simulink model "new_photovoltaic_battery_commonload"  (R2022b)
settings: Solver=FixedStepAuto  StartTime=0  StopTime=2.4  FixedStep=2e-5  RelTol=1e-3
undefined symbols (not defined in the file): Acid, Lead, sigbuilder_block
libraries: spsMeanLib x22, spsVoltageMeasurementLib x19, spsCurrentMeasurementLib x16, spsGroundLib x15, spsIdealSwitchLib x12, spsSeriesRLCLoadLib x12, spsSeriesRLCBranchLib x5, simulink x4, spsThreePhaseVIMeasurementLib x4, spsThreePhaseSeriesRLCBranchLib x2, spsThreePhaseBreakerLib x2, slpidlib x2
(part 2 of 2)

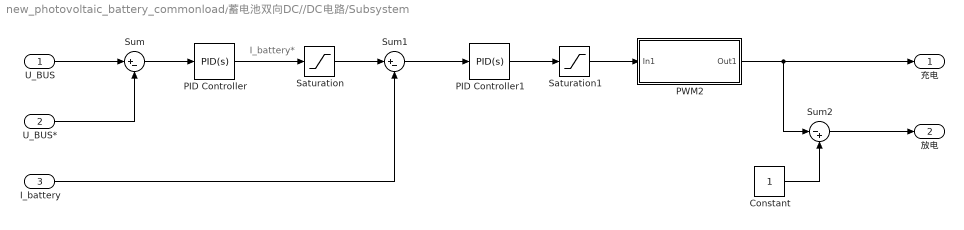
== system new_photovoltaic_battery_commonload/蓄电池双向DC//DC电路/Subsystem ==
  note: I_battery*
  U_BUS : Inport
  U_BUS* : Inport  Port=2
  I_battery : Inport  Port=3
  Constant : Constant
  PID Controller : slpidlib/PID Controller  Controller=PID  Form=Parallel  TimeDomain=Continuous-time  UseExternalTs=off  SampleTime=-1  IntegratorMethod=Forward Euler  FilterMethod=Forward Euler  ControllerParametersSource=internal  P=0.1  I=1  UseKiTs=off  D=0  N=100  UseFilter=on  TunerSelectOption=Transfer Function Based (PID Tuner App)  InitialConditionSource=internal  InitialConditionForIntegrator=0  InitialConditionForFilter=0  DifferentiatorICPrevScaledInput=0  ExternalReset=none  TrackingMode=off  Kt=1  LimitOutput=off  SatLimitsSource=internal  UpperSaturationLimit=inf  LowerSaturationLimit=-inf  LinearizeAsGain=on  AntiWindupMode=none  Kb=1  LimitIntegrator=off  UpperIntegratorSaturationLimit=inf  LowerIntegratorSaturationLimit=-inf  POutMin=[]  POutMax=[]  IOutMin=[]  IOutMax=[]  DOutMin=[]  DOutMax=[]  NOutMin=[]  NOutMax=[]  SumOutMin=[]  SumOutMax=[]  SaturationOutMin=[]  SaturationOutMax=[]  PParamMin=[]  PParamMax=[]  IParamMin=[]  IParamMax=[]  DParamMin=[]  DParamMax=[]  NParamMin=[]  NParamMax=[]  KbParamMin=[]  KbParamMax=[]  KtParamMin=[]  KtParamMax=[]  KbOutMin=[]  KbOutMax=[]  KtOutMin=[]  KtOutMax=[]  IntegratorOutMin=[]  IntegratorOutMax=[]  FilterOutMin=[]  FilterOutMax=[]  SumI1OutMin=[]  SumI1OutMax=[]  SumI2OutMin=[]  SumI2OutMax=[]  SumI3OutMin=[]  SumI3OutMax=[]  SumI4OutMin=[]  SumI4OutMax=[]  SumDOutMin=[]  SumDOutMax=[]  DifferentiatorOutMin=[]  DifferentiatorOutMax=[]  FilterDiffOutCoefMin=[]  FilterDiffOutCoefMax=[]  ReciprocalOutMin=[]  ReciprocalOutMax=[]  SumDenOutMin=[]  SumDenOutMax=[]  SumNumOutMin=[]  SumNumOutMax=[]  DivideOutMin=[]  DivideOutMax=[]  UdiffTsProdOutMin=[]  UdiffTsProdOutMax=[]  NTsProdOutMin=[]  NTsProdOutMax=[]  UintegralTsProdOutMin=[]  UintegralTsProdOutMax=[]  UngainTsProdOutMin=[]  UngainTsProdOutMax=[]  ClampingZeroOutDataTypeStr=Inherit: Inherit via back propagation  ClampingZeroOutMin=[]  ClampingZeroOutMax=[]  FilterDenConstantOutDataTypeStr=Inherit: Inherit via back propagation  FilterDenConstantOutMin=[]  FilterDenConstantOutMax=[]  PCopyOutDataTypeStr=Inherit: Inherit via back propagation  PCopyOutMin=[]  PCopyOutMax=[]  NCopyOutDataTypeStr=Inherit: Inherit via back propagation  NCopyOutMin=[]  NCopyOutMax=[]  IntegratorContinuousStateAttributes=''  IntegratorStateMustResolveToSignalObject=off  IntegratorRTWStateStorageClass=Auto  FilterContinuousStateAttributes=''  FilterStateMustResolveToSignalObject=off  FilterRTWStateStorageClass=Auto  ParallelPVariant=InternalParameters  IdealPVariant=Disabled  IVariant=InternalParameters  DVariant=InternalParameters  IntegratorVariant=Continuous  SatVariant=Disabled  AWVariant=Passthrough  PCopyVariant=Disabled  TRVariant=Disabled  FdbkBlocksVariant=Forward  IdealPFdbkVariant=Disabled  SatFdbkVariant=Disabled  DerivativeFilterVariant=ContFilter  NVariant=InternalParameters  NCopyVariant=Disabled  FilterICVariant=InternalICsFilter  IntegratorICVariant=InternalICs  ExternalResetVariant=Disabled  TRSumVariant=Passthrough  SumFdbkVariant=Disabled  SumVariant=Sum_PID  TsampFilterVariant=InternalTs  TsampNgainVariant=Passthrough  TsampIntegralVariant=Passthrough  ExternalSaturationOutDataTypeStr=Inherit: Same as second input
  PID Controller1 : slpidlib/PID Controller  Controller=PID  Form=Parallel  TimeDomain=Continuous-time  UseExternalTs=off  SampleTime=-1  IntegratorMethod=Forward Euler  FilterMethod=Forward Euler  ControllerParametersSource=internal  P=0.02  I=1  UseKiTs=off  D=0  N=100  UseFilter=on  TunerSelectOption=Transfer Function Based (PID Tuner App)  InitialConditionSource=internal  InitialConditionForIntegrator=0  InitialConditionForFilter=0  DifferentiatorICPrevScaledInput=0  ExternalReset=none  TrackingMode=off  Kt=1  LimitOutput=off  SatLimitsSource=internal  UpperSaturationLimit=inf  LowerSaturationLimit=-inf  LinearizeAsGain=on  AntiWindupMode=none  Kb=1  LimitIntegrator=off  UpperIntegratorSaturationLimit=inf  LowerIntegratorSaturationLimit=-inf  POutMin=[]  POutMax=[]  IOutMin=[]  IOutMax=[]  DOutMin=[]  DOutMax=[]  NOutMin=[]  NOutMax=[]  SumOutMin=[]  SumOutMax=[]  SaturationOutMin=[]  SaturationOutMax=[]  PParamMin=[]  PParamMax=[]  IParamMin=[]  IParamMax=[]  DParamMin=[]  DParamMax=[]  NParamMin=[]  NParamMax=[]  KbParamMin=[]  KbParamMax=[]  KtParamMin=[]  KtParamMax=[]  KbOutMin=[]  KbOutMax=[]  KtOutMin=[]  KtOutMax=[]  IntegratorOutMin=[]  IntegratorOutMax=[]  FilterOutMin=[]  FilterOutMax=[]  SumI1OutMin=[]  SumI1OutMax=[]  SumI2OutMin=[]  SumI2OutMax=[]  SumI3OutMin=[]  SumI3OutMax=[]  SumI4OutMin=[]  SumI4OutMax=[]  SumDOutMin=[]  SumDOutMax=[]  DifferentiatorOutMin=[]  DifferentiatorOutMax=[]  FilterDiffOutCoefMin=[]  FilterDiffOutCoefMax=[]  ReciprocalOutMin=[]  ReciprocalOutMax=[]  SumDenOutMin=[]  SumDenOutMax=[]  SumNumOutMin=[]  SumNumOutMax=[]  DivideOutMin=[]  DivideOutMax=[]  UdiffTsProdOutMin=[]  UdiffTsProdOutMax=[]  NTsProdOutMin=[]  NTsProdOutMax=[]  UintegralTsProdOutMin=[]  UintegralTsProdOutMax=[]  UngainTsProdOutMin=[]  UngainTsProdOutMax=[]  ClampingZeroOutDataTypeStr=Inherit: Inherit via back propagation  ClampingZeroOutMin=[]  ClampingZeroOutMax=[]  FilterDenConstantOutDataTypeStr=Inherit: Inherit via back propagation  FilterDenConstantOutMin=[]  FilterDenConstantOutMax=[]  PCopyOutDataTypeStr=Inherit: Inherit via back propagation  PCopyOutMin=[]  PCopyOutMax=[]  NCopyOutDataTypeStr=Inherit: Inherit via back propagation  NCopyOutMin=[]  NCopyOutMax=[]  IntegratorContinuousStateAttributes=''  IntegratorStateMustResolveToSignalObject=off  IntegratorRTWStateStorageClass=Auto  FilterContinuousStateAttributes=''  FilterStateMustResolveToSignalObject=off  FilterRTWStateStorageClass=Auto  ParallelPVariant=InternalParameters  IdealPVariant=Disabled  IVariant=InternalParameters  DVariant=InternalParameters  IntegratorVariant=Continuous  SatVariant=Disabled  AWVariant=Passthrough  PCopyVariant=Disabled  TRVariant=Disabled  FdbkBlocksVariant=Forward  IdealPFdbkVariant=Disabled  SatFdbkVariant=Disabled  DerivativeFilterVariant=ContFilter  NVariant=InternalParameters  NCopyVariant=Disabled  FilterICVariant=InternalICsFilter  IntegratorICVariant=InternalICs  ExternalResetVariant=Disabled  TRSumVariant=Passthrough  SumFdbkVariant=Disabled  SumVariant=Sum_PID  TsampFilterVariant=InternalTs  TsampNgainVariant=Passthrough  TsampIntegralVariant=Passthrough  ExternalSaturationOutDataTypeStr=Inherit: Same as second input
  PWM2 : Subsystem
  Saturation : Saturate  UpperLimit=40  LowerLimit=-40
  Saturation1 : Saturate  UpperLimit=0.95  LowerLimit=0.05
  Sum : Sum  Inputs=|+-
  Sum1 : Sum  Inputs=|+-
  Sum2 : Sum  Inputs=|-+
  充电 : Outport
  放电 : Outport  Port=2
  wires:
  U_BUS/1 -> Sum/1
  U_BUS*/1 -> Sum/2
  PID Controller/1 -> Saturation/1
  Sum/1 -> PID Controller/1
  Saturation/1 -> Sum1/1
  I_battery/1 -> Sum1/2
  Sum1/1 -> PID Controller1/1
  PID Controller1/1 -> Saturation1/1
  Constant/1 -> Sum2/2
  PWM2/1(Out1) -> Sum2/1, 充电/1
  Sum2/1 -> 放电/1
  Saturation1/1 -> PWM2/1(In1)

== system new_photovoltaic_battery_commonload/蓄电池双向DC//DC电路/Subsystem/PWM2 ==
  In1 : Inport
  Constant : Constant
  Constant1 : Constant  Value=0
  Repeating Sequence : simulink/Sources/Repeating Sequence  rep_seq_t=[0 1e-4]  rep_seq_y=[0 2]
  Saturation : Saturate  UpperLimit=1  LowerLimit=0
  Scope : Scope  NumInputPorts=2
  Sum : Sum  Inputs=|+-
  Switch : Switch  Criteria=u2 > Threshold  SaturateOnIntegerOverflow=off  InputSameDT=off
  Zero-Order Hold : ZeroOrderHold  SampleTime=0.05
  Out1 : Outport
  wires:
  In1/1 -> Zero-Order Hold/1
  Zero-Order Hold/1 -> Saturation/1
  Switch/1 -> Scope/1, Out1/1
  Constant/1 -> Switch/1
  Constant1/1 -> Switch/3
  Saturation/1 -> Sum/1
  Sum/1 -> Switch/2
  Repeating Sequence/1 -> Scope/2, Sum/2

== matlab function new_photovoltaic_battery_commonload/新负荷1/电灯的使用曲线 input:当前时间点 output:开启状态 ==
  data: u input; y output
function y = fcn(u)
    if u>0.6&&u<2.1
        y=1;
    else
        y=0;
    end
end

== matlab function new_photovoltaic_battery_commonload/新负荷1/电饭锅的使用曲线 input:当前时间点 output:开启状态 ==
  data: u input; y output
function y = fcn(u)
    if u>1.9&&u<2.1
        y=1;
    else
        y=0;
    end
end

== matlab function new_photovoltaic_battery_commonload/新负荷1/空调的使用曲线 input:当前时间点 output:开启状态 ==
  data: u input; y output
function y = fcn(u)
    if u>1.5&&u<2.1
        y=1;
    else
        y=0;
    end
end

== matlab function new_photovoltaic_battery_commonload/新负荷2/洗衣机的使用曲线 input:当前时间点 output:开启状态 ==
  data: u input; y output
function y = fcn(u)
    if u>1.0&&u<2.1
        y=1;
    else
        y=0;
    end
end

== matlab function new_photovoltaic_battery_commonload/新负荷2/电灯的使用曲线 input:当前时间点 output:开启状态 ==
  data: u input; y output
function y = fcn(u)
    if u>0.6&&u<2.1
        y=1;
    else
        y=0;
    end
end

== matlab function new_photovoltaic_battery_commonload/新负荷2/电饭锅的使用曲线 input:当前时间点 output:开启状态 ==
  data: u input; y output
function y = fcn(u)
    if u>1.9&&u<2.1
        y=1;
    else
        y=0;
    end
end

== matlab function new_photovoltaic_battery_commonload/新负荷2/空调的使用曲线 input:当前时间点 output:开启状态 ==
  data: u input; y output
function y = fcn(u)
    if u>1.5&&u<2.1
        y=1;
    else
        y=0;
    end
end

== matlab function new_photovoltaic_battery_commonload/新负荷/洗衣机的使用曲线 input:当前时间点 output:开启状态 ==
  data: u input; y output
function y = fcn(u)
    if u>1.0&&u<2.1
        y=1;
    else
        y=0;
    end
end

== matlab function new_photovoltaic_battery_commonload/新负荷1/洗衣机的使用曲线 input:当前时间点 output:开启状态 ==
  data: u input; y output
function y = fcn(u)
    if u>1.0&&u<2.1
        y=1;
    else
        y=0;
    end
end

== matlab function new_photovoltaic_battery_commonload/新负荷/电灯的使用曲线 input:当前时间点 output:开启状态 ==
  data: u input; y output
function y = fcn(u)
    if u>0.6&&u<2.1
        y=1;
    else
        y=0;
    end
end

== matlab function new_photovoltaic_battery_commonload/新负荷/电饭锅的使用曲线 input:当前时间点 output:开启状态 ==
  data: u input; y output
function y = fcn(u)
    if u>1.9&&u<2.1
        y=1;
    else
        y=0;
    end
end

== matlab function new_photovoltaic_battery_commonload/新负荷/空调的使用曲线 input:当前时间点 output:开启状态 ==
  data: u input; y output
function y = fcn(u)
    if u>1.5&&u<2.1
        y=1;
    else
        y=0;
    end
end
